simulink model "Receive_Realsense"  (R2024a)
settings: Solver=VariableStepAuto  StartTime=0.0  StopTime=inf  FixedStep=0.02  RelTol=1e-3
undefined symbols (not defined in the file or in its folder): Camera, gray, Standard_Devices
libraries: sldrtlib x2
settings Model: SimulationMode=accelerator  Creator=LG gram 17 - HW dev  LastModifiedBy=LG gram 17 - HW dev
settings HardwareCC: ProdBitPerLong=64  ProdHWDeviceType=Intel->x86-64 (Linux 64)
settings RTWCC: Description=Simulink Desktop Real-Time  SystemTargetFile=sldrt.tlc  TemplateMakefile=sldrt.tmf  TargetLang=C++  RTWCompilerOptimization=on  GPUComputeCapability=3.5
settings CodeAppCC: MaxIdLength=95
settings SimulinkDesktopRealTimeCC: TargetLibSuffix=_sldrt.a  TargetPreCompLibLocation=C:\Program Files\MATLAB\R2024a\toolbox\sldrt\lib\win64  TargetLangStandard=C++11 (ISO)

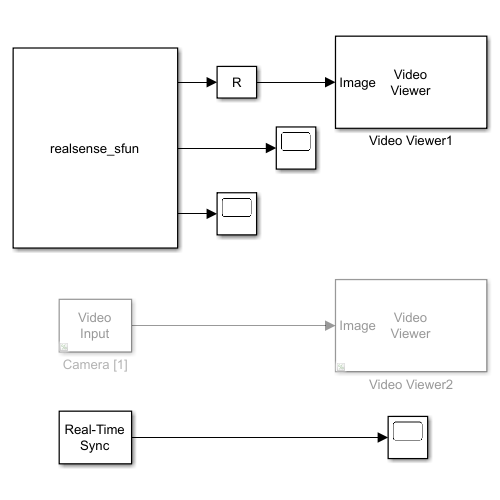
[thumbnail: Simulink's stored preview of the top-level diagram]
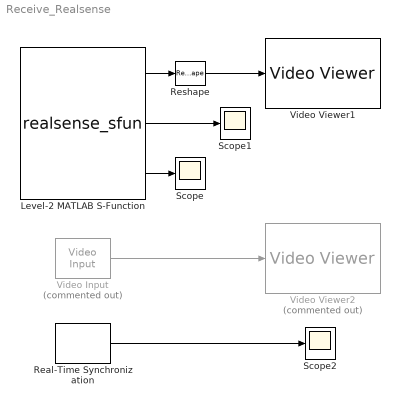
== system Receive_Realsense ==
  Level-2 MATLAB S-Function : M-S-Function  FunctionName=realsense_sfun
  Real-Time Synchronization : sldrtlib/Real-Time Synchronization  SampleTime=0.02  MaxMissedTicks=inf  ShowMissedTicks=on  YieldWhenWaiting=off
  Reshape : Reshape  OutputDimensionality=Customize  OutputDimensions=[480, 640, 3]
  Scope : Scope
  Scope1 : Scope
  Scope2 : Scope
  Video Input : sldrtlib/Video Input  Commented=on  SampleTime=0.1  MaxMissedTicks=10  ShowMissedTicks=off  YieldWhenWaiting=off  DrvName=Standard_Devices/Camera  DrvAddress=1  DrvOptions=[640 480 1]  Channels=[1 2 3]  RoiOriginSource=1  RoiOrigin=[1 1]  RoiDimensions=[640 480]  ShowReady=off  ShowError=off  ShowTimestamp=off
      settings: AttributesFormatString=Camera [1]
  Video Viewer1 : VideoViewer  colormapValue=gray(256)  FigPos=[851.666666666667 690 675.333333333333 398]
  Video Viewer2 : VideoViewer  Commented=on  colormapValue=gray(256)  FigPos=[851.666666666667 690 675.333333333333 398]
  wires:
  Level-2 MATLAB S-Function/3 -> Scope/1
  Level-2 MATLAB S-Function/2 -> Scope1/1
  Level-2 MATLAB S-Function/1 -> Reshape/1
  Reshape/1 -> Video Viewer1/1
  Video Input/1 -> Video Viewer2/1
  Real-Time Synchronization/1 -> Scope2/1
